simulink model "capstone"  (R2017b)
settings: Solver=FixedStepAuto  StartTime=0.0  StopTime=time(end)-time(1)  FixedStep=0.02  RelTol=1e-3
values from neighbouring files (symbols this model uses):
  m = 1080    [HM_SystemIdent.m]    (also in LS_SystemIdent.m = 1736.35; sumseq.m = 1)
  r = 0.335    [HM_SystemIdent.m]    (also in LS_SystemIdent.m = 0.2413)
libraries: simulink x2
settings Model: DevelopmentMode=FunctionDevelopment  OptimizingMode=Automatic  Creator=E0NF5DX  LastModifiedBy=E0NF5DX

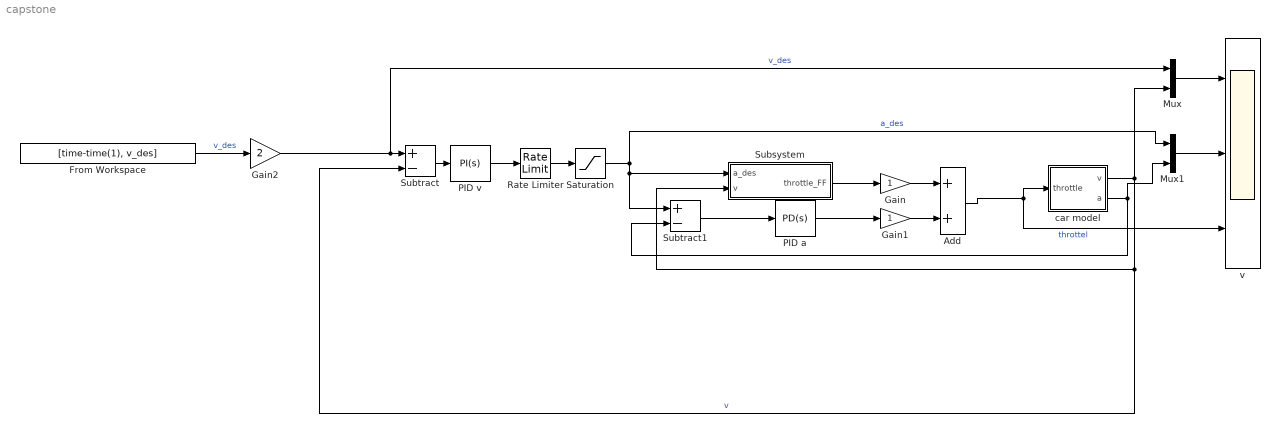
== system capstone ==
  Add : Sum
  From Workspace : FromWorkspace  VariableName=[time-time(1), v_des]  SampleTime=0
  Gain : Gain
  Gain1 : Gain
  Gain2 : Gain  Gain=2
  Mux : Mux  Inputs=2
  Mux1 : Mux  Inputs=2
  PID a : simulink/Continuous/PID Controller  Controller=PD  TimeDomain=Continuous-time  SampleTime=-1  IntegratorMethod=Forward Euler  FilterMethod=Forward Euler  Form=Parallel  UseFilter=on  ControllerParametersSource=internal  P=0.214019499899719  I=0.679932433456754  D=0  N=100  InitialConditionSource=internal  InitialConditionForIntegrator=0  InitialConditionForFilter=0  ExternalReset=none  LimitOutput=on  UpperSaturationLimit=1  LowerSaturationLimit=-5  LinearizeAsGain=on  AntiWindupMode=clamping  Kb=1  TrackingMode=off  Kt=1  PParamMin=[]  PParamMax=[]  IParamMin=[]  IParamMax=[]  DParamMin=[]  DParamMax=[]  NParamMin=[]  NParamMax=[]  KbParamMin=[]  KbParamMax=[]  KtParamMin=[]  KtParamMax=[]  POutMin=[]  POutMax=[]  IOutMin=[]  IOutMax=[]  DOutMin=[]  DOutMax=[]  NOutMin=[]  NOutMax=[]  KbOutMin=[]  KbOutMax=[]  KtOutMin=[]  KtOutMax=[]  IntegratorOutMin=[]  IntegratorOutMax=[]  FilterOutMin=[]  FilterOutMax=[]  SumOutMin=[]  SumOutMax=[]  SumI1OutMin=[]  SumI1OutMax=[]  SumI2OutMin=[]  SumI2OutMax=[]  SumI3OutMin=[]  SumI3OutMax=[]  SumDOutMin=[]  SumDOutMax=[]  SaturationOutMin=[]  SaturationOutMax=[]  IntegratorContinuousStateAttributes=''  IntegratorStateMustResolveToSignalObject=off  IntegratorRTWStateStorageClass=Auto  FilterContinuousStateAttributes=''  FilterStateMustResolveToSignalObject=off  FilterRTWStateStorageClass=Auto  DifferentiatorICPrevScaledInput=0  DifferentiatorOutMin=[]  DifferentiatorOutMax=[]  InitialConditionSetting=State (most efficient)  FilterDiffOutCoefMin=[]  FilterDiffOutCoefMax=[]  SumDenOutMin=[]  SumDenOutMax=[]  SumNumOutMin=[]  SumNumOutMax=[]  ReciprocalOutMin=[]  ReciprocalOutMax=[]  DivideOutMin=[]  DivideOutMax=[]  TunerSelectOption=Transfer Function Based (PID Tuner App)
  PID v : simulink/Continuous/PID Controller  Controller=PI  TimeDomain=Continuous-time  SampleTime=-1  IntegratorMethod=Forward Euler  FilterMethod=Forward Euler  Form=Parallel  UseFilter=on  ControllerParametersSource=internal  P=3.34015153159759  I=0.195063315771896  D=-0.267252788824667  N=19.9729001739592  InitialConditionSource=internal  InitialConditionForIntegrator=0  InitialConditionForFilter=0  ExternalReset=none  LimitOutput=on  UpperSaturationLimit=1  LowerSaturationLimit=-5  LinearizeAsGain=on  AntiWindupMode=clamping  Kb=1  TrackingMode=off  Kt=1  PParamMin=[]  PParamMax=[]  IParamMin=[]  IParamMax=[]  DParamMin=[]  DParamMax=[]  NParamMin=[]  NParamMax=[]  KbParamMin=[]  KbParamMax=[]  KtParamMin=[]  KtParamMax=[]  POutMin=[]  POutMax=[]  IOutMin=[]  IOutMax=[]  DOutMin=[]  DOutMax=[]  NOutMin=[]  NOutMax=[]  KbOutMin=[]  KbOutMax=[]  KtOutMin=[]  KtOutMax=[]  IntegratorOutMin=[]  IntegratorOutMax=[]  FilterOutMin=[]  FilterOutMax=[]  SumOutMin=[]  SumOutMax=[]  SumI1OutMin=[]  SumI1OutMax=[]  SumI2OutMin=[]  SumI2OutMax=[]  SumI3OutMin=[]  SumI3OutMax=[]  SumDOutMin=[]  SumDOutMax=[]  SaturationOutMin=[]  SaturationOutMax=[]  IntegratorContinuousStateAttributes=''  IntegratorStateMustResolveToSignalObject=off  IntegratorRTWStateStorageClass=Auto  FilterContinuousStateAttributes=''  FilterStateMustResolveToSignalObject=off  FilterRTWStateStorageClass=Auto  DifferentiatorICPrevScaledInput=0  DifferentiatorOutMin=[]  DifferentiatorOutMax=[]  InitialConditionSetting=State (most efficient)  FilterDiffOutCoefMin=[]  FilterDiffOutCoefMax=[]  SumDenOutMin=[]  SumDenOutMax=[]  SumNumOutMin=[]  SumNumOutMax=[]  ReciprocalOutMin=[]  ReciprocalOutMax=[]  DivideOutMin=[]  DivideOutMax=[]  TunerSelectOption=Transfer Function Based (PID Tuner App)
  Rate Limiter : RateLimiter  RisingSlewLimit=10  FallingSlewLimit=-10  SampleTimeMode=inherited
  Saturation : Saturate  UpperLimit=1  LowerLimit=-5
  Subsystem : Subsystem
  Subtract : Sum  Inputs=+-  RndMeth=Zero  InputSameDT=on  OutDataTypeStr=Inherit: Same as first input
  Subtract1 : Sum  Inputs=+-  RndMeth=Zero  InputSameDT=on  OutDataTypeStr=Inherit: Same as first input
  car model : Subsystem
  v : Scope  NumInputPorts=3
  wires:
  Gain2/1 -> Mux/1, Subtract/1  "v_des"
  car model/1(v) -> Subsystem/2(v), Subtract/2, Mux/2  "v"
  Subtract/1 -> PID v/1
  PID v/1 -> Rate Limiter/1
  Mux/1 -> v/1
  Rate Limiter/1 -> Saturation/1
  Saturation/1 -> Subsystem/1(a_des), Subtract1/1, Mux1/1  "a_des"
  car model/2(a) -> Subtract1/2, Mux1/2
  Subtract1/1 -> PID a/1
  Add/1 -> v/3, car model/1(throttle)  "throttel"
  Mux1/1 -> v/2
  Subsystem/1(throttle_FF) -> Gain/1
  PID a/1 -> Gain1/1
  Gain/1 -> Add/1
  Gain1/1 -> Add/2
  From Workspace/1 -> Gain2/1  "v_des"

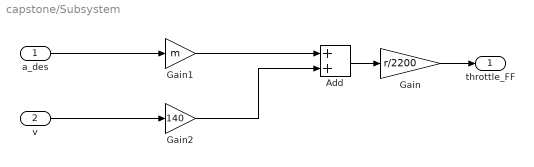
== system capstone/Subsystem ==
  a_des : Inport
  v : Inport  Port=2
  Add : Sum
  Gain : Gain  Gain=r/2200  RndMeth=Zero  OutDataTypeStr=Inherit: Same as input  ParamDataTypeStr=Inherit: Same as input
  Gain1 : Gain  Gain=m  RndMeth=Zero  OutDataTypeStr=Inherit: Same as input  ParamDataTypeStr=Inherit: Same as input
  Gain2 : Gain  Gain=140  RndMeth=Zero  OutDataTypeStr=Inherit: Same as input  ParamDataTypeStr=Inherit: Same as input
  throttle_FF : Outport
  wires:
  Gain/1 -> throttle_FF/1
  Add/1 -> Gain/1
  a_des/1 -> Gain1/1
  Gain1/1 -> Add/1
  v/1 -> Gain2/1
  Gain2/1 -> Add/2

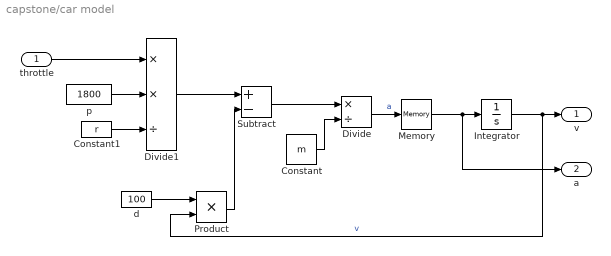
== system capstone/car model ==
  throttle : Inport
      settings: AttributesFormatString=<[%<OutMin> %<OutMax>]>
  Constant : Constant  Value=m
  Constant1 : Constant  Value=r
  Divide : Product  Inputs=*/  RndMeth=Zero  InputSameDT=on  OutDataTypeStr=Inherit: Same as first input
  Divide1 : Product  Inputs=**/  RndMeth=Zero  InputSameDT=on  OutDataTypeStr=Inherit: Same as first input
  Integrator : Integrator
  Memory : Memory
  Product : Product  RndMeth=Zero  InputSameDT=on  OutDataTypeStr=Inherit: Same as first input
  Subtract : Sum  Inputs=+-  RndMeth=Zero  InputSameDT=on  OutDataTypeStr=Inherit: Same as first input
  d : Constant  Value=100
  p : Constant  Value=1800
  v : Outport
      settings: AttributesFormatString=<[%<OutMin> %<OutMax>]; %<OutputWhenDisabled>>
  a : Outport  Port=2
      settings: AttributesFormatString=<[%<OutMin> %<OutMax>]; %<OutputWhenDisabled>>
  wires:
  Divide/1 -> Memory/1  "a"
  Constant/1 -> Divide/2
  Subtract/1 -> Divide/1
  throttle/1 -> Divide1/1
  p/1 -> Divide1/2
  Constant1/1 -> Divide1/3
  Divide1/1 -> Subtract/1
  Product/1 -> Subtract/2
  d/1 -> Product/1
  Integrator/1 -> Product/2, v/1  "v"
  Memory/1 -> a/1, Integrator/1
